simulink model "BEVplantModel"  (R2022b)
settings: Solver=daessc  StartTime=0  StopTime=50  RelTol=1e-3
PreLoadFcn:
  | % Load all parameters
  | BEVplantModelParam;
undefined symbols (not defined in the file): battery, cabin_T_init, coolant_pipe_D, coolant_valve_D_ratio_max, coolant_valve_D_ratio_min, coolant_valve_displacement, electricDrive, max_torque, vehicle, vehicleThermal
libraries: fl_lib x292, nesl_utility x67, SimscapeFluids_lib x15, ee_lib x11, sdl_lib x8, BatteryCurrentManagement x3, slpidlib x3, simulink x2, BatteryThermalManagement x1, autolibshared x1
(part 6 of 10)

== system BEVplantModel/Vehicle/Front Motor (EM1)/Inverter Power Module Thermal ==
  PM Cauer thermall : Subsystem
      settings: PortSchema="{\"entries\":[{\"content\":{\"sides\":[{\"content\":{\"connectorIds\":[\"LConn1\",\"Out1\",\"Out2\"]},\"type\":\"ConnectorPlacement.EquallySpacedRectSide\",\"uuid\":\"c466717f-a559-4c42-b6dd-2de508982627\"},{\"content\":{\"connectorIds\":[\"RConn1\",\"RConn2\"],\"side\":\"RIGHT\"},\"type\":\"ConnectorPlacement.EquallySpacedRectSide\",\"uuid\":\"5a44429a-0c01-47a4-96c4-89a03d92af2a\"},{\"content\":{\"connectorIds\":[],\"side\":\"TOP\"},\"type\":\"ConnectorPlacement.EquallySpacedRectSide\",\"uuid\":\"592797f6-2176-45a1-8a5a-ffba72eaaa30\"},{\"content\":{\"connectorIds\":[\"RConn3\"],\"side\":\"BOTTOM\"},\"type\":\"ConnectorPlacement.EquallySpacedRectSide\",\"uuid\":\"45f39216-5c54-48d4-857b-159bfbffda40\"}]},\"type\":\"ConnectorPlacement.EquallySpacedConnector\",\"uuid\":\"8211d252-7bec-4c59-be39-60a0fcf206ce\"}],\"packageUris\":[\"http://schema.mathworks.com/mf0/Connector/R2020b\"],\"version\":\"1.0\"}"
  PS Lookup Table (3D)1 : fl_lib/Physical Signals/Lookup Tables/PS Lookup Table (3D)  x1=electricDrive.loss_maps.spMat rpm  x2=electricDrive.loss_maps.tqMat N*m  x3=[25,125, 175]+273.15 K  f=electricDrive.loss_maps_inv.lossMatIgbt  interp_method=simscape.enum.interpolation.linear  extrap_method=simscape.enum.extrapolation.linear
      settings: InternalSimscapePortConfiguration="{\"Bottom\":[],\"Left\":[{\"id\":\"I1\",\"label\":\"x1\",\"type\":\"input\"},{\"id\":\"I2\",\"label\":\"x2\",\"type\":\"input\"},{\"id\":\"I3\",\"label\":\"x3\",\"type\":\"input\"}],\"Right\":[{\"id\":\"O\",\"label\":\"f\",\"type\":\"output\"}],\"Top\":[]}"
  PS Lookup Table (3D)2 : fl_lib/Physical Signals/Lookup Tables/PS Lookup Table (3D)  x1=electricDrive.loss_maps.spMat rpm  x2=electricDrive.loss_maps.tqMat N*m  x3=[25,125, 175]+273.15 K  f=electricDrive.loss_maps_inv.lossMatDiode  interp_method=simscape.enum.interpolation.linear  extrap_method=simscape.enum.extrapolation.linear
      settings: InternalSimscapePortConfiguration="{\"Bottom\":[],\"Left\":[{\"id\":\"I1\",\"label\":\"x1\",\"type\":\"input\"},{\"id\":\"I2\",\"label\":\"x2\",\"type\":\"input\"},{\"id\":\"I3\",\"label\":\"x3\",\"type\":\"input\"}],\"Right\":[{\"id\":\"O\",\"label\":\"f\",\"type\":\"output\"}],\"Top\":[]}"
  Simulink-PS Converter : nesl_utility/Simulink-PS Converter  PhysicalDomain=network_engine_domain  SubClassName=ps_input  LeftPortType=input  RightPortType=output  PseudoPeriodic=off  Frequencies=[]  NoiseDistribution=none  NoiseParameters=[]  Unit=K  AffineConversion=off  FilteringAndDerivatives=provide  SimscapeFilterOrder=1  InputFilterTimeConstant=0.001  UdotUserProvided=0
  Simulink-PS Converter1 : nesl_utility/Simulink-PS Converter  PhysicalDomain=network_engine_domain  SubClassName=ps_input  LeftPortType=input  RightPortType=output  PseudoPeriodic=off  Frequencies=[]  NoiseDistribution=none  NoiseParameters=[]  Unit=K  AffineConversion=off  FilteringAndDerivatives=provide  SimscapeFilterOrder=1  InputFilterTimeConstant=0.001  UdotUserProvided=0
  Vliq : PMIOPort  Side=Left
  Motor RPM : PMIOPort  Port=2  Side=Left
  Motor Torque : PMIOPort  Port=3  Side=Left
  H : PMIOPort  Port=4  Side=Right
  wires:
  PM Cauer thermall/1(IGBT) -> [Tigbt]
  PM Cauer thermall/2(Diode) -> [Tdiode]
  [Tdiode] -> Simulink-PS Converter1/1
  [Tigbt] -> Simulink-PS Converter/1
  connections:
  H/RConn1 -- PM Cauer thermall/LConn1
  PS Lookup Table (3D)1/RConn1 -- PM Cauer thermall/RConn2
  PS Lookup Table (3D)2/RConn1 -- PM Cauer thermall/RConn1
  Vliq/RConn1 -- PM Cauer thermall/RConn3
  Motor RPM/RConn1 -- PS Lookup Table (3D)1/LConn1 -- PS Lookup Table (3D)2/LConn1
  Motor Torque/RConn1 -- PS Lookup Table (3D)1/LConn2 -- PS Lookup Table (3D)2/LConn2
  Simulink-PS Converter1/RConn1 -- PS Lookup Table (3D)2/LConn3
  Simulink-PS Converter/RConn1 -- PS Lookup Table (3D)1/LConn3

== system BEVplantModel/Vehicle/Front Motor (EM1)/SC1 ==
  Absolute Reference (TL) : fl_lib/Thermal Liquid/Elements/Absolute Reference (TL)
  Pressure & Temperature Sensor (TL) : fl_lib/Thermal Liquid/Sensors/Pressure & Temperature Sensor (TL)
      settings: InternalSimscapePortConfiguration="{\"Bottom\":[],\"Left\":[{\"id\":\"A\",\"label\":\"A\",\"type\":\"foundation.thermal_liquid.thermal_liquid\"}],\"Right\":[{\"id\":\"B\",\"label\":\"B\",\"type\":\"foundation.thermal_liquid.thermal_liquid\"},{\"id\":\"P\",\"label\":\"P\",\"type\":\"output\"},{\"id\":\"T\",\"label\":\"T\",\"type\":\"output\"}],\"Top\":[]}"
  Volumetric Flow Rate Sensor (TL) : fl_lib/Thermal Liquid/Sensors/Volumetric Flow Rate Sensor (TL)
      settings: InternalSimscapePortConfiguration="{\"Bottom\":[],\"Left\":[{\"id\":\"A\",\"label\":\"A\",\"type\":\"foundation.thermal_liquid.thermal_liquid\"}],\"Right\":[{\"id\":\"B\",\"label\":\"B\",\"type\":\"foundation.thermal_liquid.thermal_liquid\"},{\"id\":\"V\",\"label\":\"V\",\"type\":\"output\"}],\"Top\":[]}"
  B : PMIOPort  Side=Left
  A : PMIOPort  Port=2  Side=Right
  m3/s : PMIOPort  Port=3  Side=Right
  connections:
  Pressure & Temperature Sensor (TL)/LConn1 -- Volumetric Flow Rate Sensor (TL)/RConn1 -- A/RConn1
  Volumetric Flow Rate Sensor (TL)/LConn1 -- B/RConn1
  Absolute Reference (TL)/LConn1 -- Pressure & Temperature Sensor (TL)/RConn1
  Volumetric Flow Rate Sensor (TL)/RConn2 -- m3/s/RConn1

== system BEVplantModel/Vehicle/Front Motor (EM1)/TempSens ==
  Absolute Reference (TL) : fl_lib/Thermal Liquid/Elements/Absolute Reference (TL)
  PS-Simulink Converter7 : nesl_utility/PS-Simulink Converter  PhysicalDomain=network_engine_domain  SubClassName=ps_output  LeftPortType=input  RightPortType=output  PseudoPeriodic=off  Frequencies=[]  VectorFormat=inherit  Unit=inherit  AffineConversion=off
  Pressure & Temperature Sensor (TL) : fl_lib/Thermal Liquid/Sensors/Pressure & Temperature Sensor (TL)
      settings: InternalSimscapePortConfiguration="{\"Bottom\":[],\"Left\":[{\"id\":\"A\",\"label\":\"A\",\"type\":\"foundation.thermal_liquid.thermal_liquid\"}],\"Right\":[{\"id\":\"B\",\"label\":\"B\",\"type\":\"foundation.thermal_liquid.thermal_liquid\"},{\"id\":\"P\",\"label\":\"P\",\"type\":\"output\"},{\"id\":\"T\",\"label\":\"T\",\"type\":\"output\"}],\"Top\":[]}"
  " " : PMIOPort  Side=Left
  "  " : Outport
  wires:
  PS-Simulink Converter7/1 -> "  "/1
  connections:
  Pressure & Temperature Sensor (TL)/RConn3 -- PS-Simulink Converter7/LConn1
  Absolute Reference (TL)/LConn1 -- Pressure & Temperature Sensor (TL)/RConn1
  Pressure & Temperature Sensor (TL)/LConn1 -- " "/RConn1

== system BEVplantModel/Vehicle/Front Motor (EM1)/m3//s to m//s ==
  note: Q=Av
  Coolant Area : fl_lib/Physical Signals/Sources/PS Constant  constant=4 * pi * vehicleThermal.coolant_channel_D^2 / 4 m^2
  PS Divide : fl_lib/Physical Signals/Functions/PS Divide
  PS Saturation : fl_lib/Physical Signals/Nonlinear Operators/PS Saturation  upper_limit=10 m/s  lower_limit=1e-6 m/s
  "  " : PMIOPort  Side=Left
  Vliq : PMIOPort  Port=2  Side=Right
  connections:
  PS Divide/LConn2 -- Coolant Area/RConn1
  "  "/RConn1 -- PS Divide/LConn1
  PS Divide/RConn1 -- PS Saturation/LConn1
  PS Saturation/RConn1 -- Vliq/RConn1

== system BEVplantModel/Vehicle/HVAC/Cabin ==
  Tenv : Inport
  Tsetpoint : Inport  Port=2
  acOnOff : Inport  Port=3
  HVAC Control : Subsystem
  HVAC Plant : Subsystem
  Cool : Outport
  PTC : Outport  Port=2
  wires:
  HVAC Plant/1(ptcTp) -> [Tptc]
  HVAC Control/2(PTC) -> PTC/1, HVAC Plant/3(cmdPTC)
  HVAC Control/1(cmdBlower) -> HVAC Plant/2(cmdBlower)
  HVAC Plant/2(CoolerTp) -> [TacVent]
  HVAC Plant/3(cabinTp) -> [Tcabin]
  [Tptc] -> HVAC Control/2(Tptc)
  HVAC Control/3(cmdCool) -> HVAC Plant/4(cmdCool), Cool/1
  [TacVent] -> HVAC Control/4(TacVent)
  [Tcabin] -> HVAC Control/3(Tcabin)
  Tsetpoint/1 -> HVAC Control/5(Tsetpoint)
  Tenv/1 -> HVAC Control/1(Tenv), HVAC Plant/1(EnvTp)
  acOnOff/1 -> HVAC Control/6(acOnOff)

== system BEVplantModel/Vehicle/HVAC/HVAC Demand ==
  No current : fl_lib/Physical Signals/Sources/PS Constant  constant=0 A
  PS Abs : fl_lib/Physical Signals/Nonlinear Operators/PS Abs
      settings: InternalSimscapePortConfiguration="{\"Bottom\":[],\"Left\":[{\"id\":\"I\",\"label\":\"\",\"type\":\"input\"}],\"Right\":[{\"id\":\"O\",\"label\":\"\",\"type\":\"output\"}],\"Top\":[]}"
  PS Add : fl_lib/Physical Signals/Functions/PS Add
  PS Add1 : fl_lib/Physical Signals/Functions/PS Add
  PS Divide : fl_lib/Physical Signals/Functions/PS Divide
  PS Switch : fl_lib/Physical Signals/Nonlinear Operators/PS Switch  Threshold=0.5
      settings: InternalSimscapePortConfiguration="{\"Bottom\":[],\"Left\":[{\"id\":\"I1\",\"label\":\"\",\"type\":\"input\"},{\"id\":\"I2\",\"label\":\"\",\"type\":\"input\"},{\"id\":\"I3\",\"label\":\"\",\"type\":\"input\"}],\"Right\":[{\"id\":\"O\",\"label\":\"\",\"type\":\"output\"}],\"Top\":[]}"
  Zero Divide Protection : fl_lib/Physical Signals/Sources/PS Constant  constant=1 V
  Volt : PMIOPort  Side=Left
  BatSt : PMIOPort  Port=2  Side=Left
  Cool : PMIOPort  Port=3  Side=Left
  I : PMIOPort  Port=4  Side=Right
  PTC : PMIOPort  Port=5  Side=Left
  connections:
  No current/RConn1 -- PS Switch/LConn3
  PS Add1/LConn1 -- Volt/RConn1
  PS Switch/LConn1 -- PS Divide/RConn1
  BatSt/RConn1 -- PS Switch/LConn2
  PS Switch/RConn1 -- I/RConn1
  PS Add1/RConn1 -- PS Divide/LConn2
  PS Add1/LConn2 -- Zero Divide Protection/RConn1
  PS Abs/RConn1 -- PS Add/LConn1
  Cool/RConn1 -- PS Abs/LConn1
  PTC/RConn1 -- PS Add/LConn2
  PS Add/RConn1 -- PS Divide/LConn1

== system BEVplantModel/Vehicle/HVAC/HVAC Energy ==
  I : Inport
  Batt : Inport  Port=2
  Bus Selector : BusSelector  OutputSignals=BattSensor.BatVolt
  Constant : Constant  Value=3600
  Divide : Product  Inputs=*/
  Integrator : Integrator
  Product : Product
  E : Outport
  wires:
  I/1 -> Product/1
  Divide/1 -> E/1
  Batt/1 -> Bus Selector/1
  Constant/1 -> Divide/2
  Integrator/1 -> Divide/1
  Product/1 -> Integrator/1
  Bus Selector/1 -> Product/2  "<BatVolt>"

== system BEVplantModel/Vehicle/Heater/Heater Subsystem ==
  Batt : Inport
  ThCtrl : Inport  Port=2
  Compare To Constant : simulink/Logic and Bit Operations/Compare To Constant  relop=>  const=0  OutDataTypeStr=boolean
  Heater Demand : Subsystem
  Max Power [W] : Gain  Gain=vehicleThermal.heaterMaxPower
  Product : Product
  Simulink-PS Converter : nesl_utility/Simulink-PS Converter  PhysicalDomain=network_engine_domain  SubClassName=ps_input  LeftPortType=input  RightPortType=output  PseudoPeriodic=off  Frequencies=[]  NoiseDistribution=none  NoiseParameters=[]  Unit=W  AffineConversion=off  FilteringAndDerivatives=provide  SimscapeFilterOrder=1  InputFilterTimeConstant=0.001  UdotUserProvided=0
  Simulink-PS Converter2 : nesl_utility/Simulink-PS Converter  PhysicalDomain=network_engine_domain  SubClassName=ps_input  LeftPortType=input  RightPortType=output  PseudoPeriodic=off  Frequencies=[]  NoiseDistribution=none  NoiseParameters=[]  Unit=1  AffineConversion=off  FilteringAndDerivatives=provide  SimscapeFilterOrder=1  InputFilterTimeConstant=0.001  UdotUserProvided=0
  Transfer Fcn : TransferFcn  Denominator=[1 1]
  V : PMIOPort  Side=Left
  I : PMIOPort  Port=2  Side=Right
  output : PMIOPort  Port=3  Side=Right
  wires:
  Product/1 -> Simulink-PS Converter/1
  Transfer Fcn/1 -> Max Power [W]/1
  Max Power [W]/1 -> Product/2
  Compare To Constant/1 -> Product/1
  ThCtrl/1 -> Transfer Fcn/1
  Batt/1 -> Compare To Constant/1, Simulink-PS Converter2/1
  connections:
  Simulink-PS Converter/RConn1 -- Heater Demand/LConn3 -- output/RConn1
  Heater Demand/LConn1 -- V/RConn1
  Heater Demand/LConn2 -- Simulink-PS Converter2/RConn1
  Heater Demand/RConn1 -- I/RConn1

== system BEVplantModel/Vehicle/Heater/current sensing1 ==
  Current Sensor : fl_lib/Electrical/Electrical Sensors/Current Sensor
  PS-Simulink Converter : nesl_utility/PS-Simulink Converter  PhysicalDomain=network_engine_domain  SubClassName=ps_output  LeftPortType=input  RightPortType=output  PseudoPeriodic=off  Frequencies=[]  VectorFormat=inherit  Unit=inherit  AffineConversion=off
  "  " : PMIOPort  Side=Left
  " " : PMIOPort  Port=2  Side=Right
  "   " : Outport
  wires:
  PS-Simulink Converter/1 -> "   "/1
  connections:
  PS-Simulink Converter/LConn1 -- Current Sensor/RConn1
  Current Sensor/LConn1 -- "  "/RConn1
  Current Sensor/RConn2 -- " "/RConn1

== system BEVplantModel/Vehicle/Motor Pump/Pump Demand ==
  No current : fl_lib/Physical Signals/Sources/PS Constant  constant=0 A
  PS Abs : fl_lib/Physical Signals/Nonlinear Operators/PS Abs
      settings: InternalSimscapePortConfiguration="{\"Bottom\":[],\"Left\":[{\"id\":\"I\",\"label\":\"\",\"type\":\"input\"}],\"Right\":[{\"id\":\"O\",\"label\":\"\",\"type\":\"output\"}],\"Top\":[]}"
  PS Divide : fl_lib/Physical Signals/Functions/PS Divide
  PS Product : fl_lib/Physical Signals/Functions/PS Product
  PS Switch : fl_lib/Physical Signals/Nonlinear Operators/PS Switch  Threshold=0.5
      settings: InternalSimscapePortConfiguration="{\"Bottom\":[],\"Left\":[{\"id\":\"I1\",\"label\":\"\",\"type\":\"input\"},{\"id\":\"I2\",\"label\":\"\",\"type\":\"input\"},{\"id\":\"I3\",\"label\":\"\",\"type\":\"input\"}],\"Right\":[{\"id\":\"O\",\"label\":\"\",\"type\":\"output\"}],\"Top\":[]}"
  PS Switch1 : fl_lib/Physical Signals/Nonlinear Operators/PS Switch  Threshold=0.5
      settings: InternalSimscapePortConfiguration="{\"Bottom\":[],\"Left\":[{\"id\":\"I1\",\"label\":\"\",\"type\":\"input\"},{\"id\":\"I2\",\"label\":\"\",\"type\":\"input\"},{\"id\":\"I3\",\"label\":\"\",\"type\":\"input\"}],\"Right\":[{\"id\":\"O\",\"label\":\"\",\"type\":\"output\"}],\"Top\":[]}"
  Zero Divide Protection : fl_lib/Physical Signals/Sources/PS Constant  constant=1 V
  BatSt : PMIOPort  Side=Left
  Volt : PMIOPort  Port=2  Side=Left
  Q : PMIOPort  Port=3  Side=Left
  P : PMIOPort  Port=4  Side=Left
  I : PMIOPort  Port=5  Side=Right
  connections:
  No current/RConn1 -- PS Switch/LConn3
  PS Switch1/LConn1 -- Volt/RConn1
  PS Switch/LConn1 -- PS Divide/RConn1
  BatSt/RConn1 -- PS Switch1/LConn2 -- PS Switch/LConn2
  PS Switch/RConn1 -- I/RConn1
  PS Divide/LConn1 -- PS Product/RConn1
  PS Abs/RConn1 -- PS Product/LConn2
  Q/RConn1 -- PS Product/LConn1
  P/RConn1 -- PS Abs/LConn1
  PS Switch1/RConn1 -- PS Divide/LConn2
  Zero Divide Protection/RConn1 -- PS Switch1/LConn3

== system BEVplantModel/Vehicle/Motor Pump/current sensing1 ==
  Current Sensor : fl_lib/Electrical/Electrical Sensors/Current Sensor
  PS-Simulink Converter : nesl_utility/PS-Simulink Converter  PhysicalDomain=network_engine_domain  SubClassName=ps_output  LeftPortType=input  RightPortType=output  PseudoPeriodic=off  Frequencies=[]  VectorFormat=inherit  Unit=inherit  AffineConversion=off
  "  " : PMIOPort  Side=Left
  " " : PMIOPort  Port=2  Side=Right
  "   " : Outport
  wires:
  PS-Simulink Converter/1 -> "   "/1
  connections:
  PS-Simulink Converter/LConn1 -- Current Sensor/RConn1
  Current Sensor/LConn1 -- "  "/RConn1
  Current Sensor/RConn2 -- " "/RConn1

== system BEVplantModel/Vehicle/Parallel-Serial Mode Valve/Battery Coolant Tank Heat Transfer ==
  Tenv : Inport
  Convective Heat Transfer : fl_lib/Thermal/Thermal Elements/Convective Heat Transfer  thermal_type=foundation.enum.constant_variable.constant  area=3 * vehicleThermal.coolant_tank_area m^2  heat_tr_coeff=20 W/(m^2 * K)  min_heat_tr_coeff=1e-3 W/(K*m^2)  T_specify=off  T_priority=None  T=0 K  T_nominal_specify=off  T_nominal_unit=K  T_nominal_value=1  Q_specify=off  Q_priority=None  Q=0 W  Q_nominal_specify=off  Q_nominal_unit=W  Q_nominal_value=1
  Convective Heat Transfer1 : fl_lib/Thermal/Thermal Elements/Convective Heat Transfer  thermal_type=foundation.enum.constant_variable.constant  area=3 * vehicleThermal.coolant_tank_area m^2  heat_tr_coeff=20 W/(m^2 * K)  min_heat_tr_coeff=1e-3 W/(K*m^2)  T_specify=off  T_priority=None  T=0 K  T_nominal_specify=off  T_nominal_unit=K  T_nominal_value=1  Q_specify=off  Q_priority=None  Q=0 W  Q_nominal_specify=off  Q_nominal_unit=W  Q_nominal_value=1
  Environment Temperature : fl_lib/Thermal/Thermal Sources/Controlled Temperature Source
  Simulink-PS Converter : nesl_utility/Simulink-PS Converter  PhysicalDomain=network_engine_domain  SubClassName=ps_input  LeftPortType=input  RightPortType=output  PseudoPeriodic=off  Frequencies=[]  NoiseDistribution=none  NoiseParameters=[]  Unit=K  AffineConversion=on  FilteringAndDerivatives=provide  SimscapeFilterOrder=1  InputFilterTimeConstant=0.001  UdotUserProvided=0
  Thermal Reference : fl_lib/Thermal/Thermal Elements/Thermal Reference
  A : PMIOPort  Side=Left
  B : PMIOPort  Port=2  Side=Left
  wires:
  Tenv/1 -> Simulink-PS Converter/1
  connections:
  Convective Heat Transfer/RConn1 -- Convective Heat Transfer1/RConn1 -- Environment Temperature/LConn1
  Thermal Reference/LConn1 -- Environment Temperature/RConn2
  Simulink-PS Converter/RConn1 -- Environment Temperature/RConn1
  B/RConn1 -- Convective Heat Transfer1/LConn1
  Convective Heat Transfer/LConn1 -- A/RConn1

== system BEVplantModel/Vehicle/Parallel-Serial Mode Valve/Motor Coolant Tank Heat Transfer ==
  Tenv : Inport
  Convective Heat Transfer : fl_lib/Thermal/Thermal Elements/Convective Heat Transfer  thermal_type=foundation.enum.constant_variable.constant  area=3 * vehicleThermal.coolant_tank_area m^2  heat_tr_coeff=20 W/(m^2 * K)  min_heat_tr_coeff=1e-3 W/(K*m^2)  T_specify=off  T_priority=None  T=0 K  T_nominal_specify=off  T_nominal_unit=K  T_nominal_value=1  Q_specify=off  Q_priority=None  Q=0 W  Q_nominal_specify=off  Q_nominal_unit=W  Q_nominal_value=1
  Convective Heat Transfer1 : fl_lib/Thermal/Thermal Elements/Convective Heat Transfer  thermal_type=foundation.enum.constant_variable.constant  area=3 * vehicleThermal.coolant_tank_area m^2  heat_tr_coeff=20 W/(m^2 * K)  min_heat_tr_coeff=1e-3 W/(K*m^2)  T_specify=off  T_priority=None  T=0 K  T_nominal_specify=off  T_nominal_unit=K  T_nominal_value=1  Q_specify=off  Q_priority=None  Q=0 W  Q_nominal_specify=off  Q_nominal_unit=W  Q_nominal_value=1
  Environment Temperature : fl_lib/Thermal/Thermal Sources/Controlled Temperature Source
  Simulink-PS Converter : nesl_utility/Simulink-PS Converter  PhysicalDomain=network_engine_domain  SubClassName=ps_input  LeftPortType=input  RightPortType=output  PseudoPeriodic=off  Frequencies=[]  NoiseDistribution=none  NoiseParameters=[]  Unit=K  AffineConversion=on  FilteringAndDerivatives=provide  SimscapeFilterOrder=1  InputFilterTimeConstant=0.001  UdotUserProvided=0
  Thermal Reference : fl_lib/Thermal/Thermal Elements/Thermal Reference
  A : PMIOPort  Side=Right
  B : PMIOPort  Port=2  Side=Right
  wires:
  Tenv/1 -> Simulink-PS Converter/1
  connections:
  Simulink-PS Converter/RConn1 -- Environment Temperature/RConn1
  Thermal Reference/LConn1 -- Environment Temperature/RConn2
  Convective Heat Transfer/RConn1 -- Environment Temperature/LConn1 -- Convective Heat Transfer1/RConn1
  B/RConn1 -- Convective Heat Transfer1/LConn1
  A/RConn1 -- Convective Heat Transfer/LConn1

== system BEVplantModel/Vehicle/Parallel-Serial Mode Valve/Valve Control ==
  Ctrl : Inport
  Bias : Bias  Bias=-1  SaturateOnIntegerOverflow=off
  Gain : Gain  Gain=2
  Max Valve Displacement [m] : Gain  Gain=vehicleThermal.coolant_valve_displacement
  Simulink-PS Converter : nesl_utility/Simulink-PS Converter  PhysicalDomain=network_engine_domain  SubClassName=ps_input  LeftPortType=input  RightPortType=output  PseudoPeriodic=off  Frequencies=[]  NoiseDistribution=none  NoiseParameters=[]  Unit=m  AffineConversion=off  FilteringAndDerivatives=provide  SimscapeFilterOrder=1  InputFilterTimeConstant=0.001  UdotUserProvided=0
  Transfer Fcn : TransferFcn  Denominator=[1 1]
  disp : PMIOPort  Side=Right
  wires:
  Bias/1 -> Max Valve Displacement [m]/1
  Gain/1 -> Bias/1
  Transfer Fcn/1 -> Gain/1
  Max Valve Displacement [m]/1 -> Simulink-PS Converter/1
  Ctrl/1 -> Transfer Fcn/1
  connections:
  Simulink-PS Converter/RConn1 -- disp/RConn1

== system BEVplantModel/Vehicle/Radiator/Fan_Control ==
  VehSpd : Inport
  FanCtrl : Inport  Port=2
  Air Speed Table [m/s] : Lookup_n-D  BreakpointsForDimension1=[0 40 90 110 150 180 198]  BreakpointsForDimension2=[0 14.4]  IndexSearchMethod=Linear search  BeginIndexSearchUsingPreviousIndexResult=on  Table=[0 0.8 2.2 2.7 3.6 4.1 4.6; 1.5 2.3 3.2 3.5 4.3 4.8 5.1]'  InternalRulePriority=Speed  RndMeth=Simplest
      settings: InputPortMap=u0,u1
  Fan Area [m^2] : Gain  Gain=vehicleThermal.fan_area
  Max Fan : Gain  Gain=14.4
  Simulink-PS Converter4 : nesl_utility/Simulink-PS Converter  PhysicalDomain=network_engine_domain  SubClassName=ps_input  LeftPortType=input  RightPortType=output  PseudoPeriodic=off  Frequencies=[]  NoiseDistribution=none  NoiseParameters=[]  Unit=m^3/s  AffineConversion=off  FilteringAndDerivatives=provide  SimscapeFilterOrder=1  InputFilterTimeConstant=0.001  UdotUserProvided=0
  Transfer Fcn : TransferFcn  Denominator=[5 1]
  disp : PMIOPort  Side=Right
  wires:
  Fan Area [m^2]/1 -> Simulink-PS Converter4/1
  VehSpd/1 -> Air Speed Table [m/s]/1
  FanCtrl/1 -> Max Fan/1
  Air Speed Table [m/s]/1 -> Transfer Fcn/1
  Transfer Fcn/1 -> Fan Area [m^2]/1
  Max Fan/1 -> Air Speed Table [m/s]/2
  connections:
  disp/RConn1 -- Simulink-PS Converter4/RConn1

== system BEVplantModel/Vehicle/Radiator/Subsystem ==
  s : Inport
  Bus Selector : BusSelector  OutputSignals=Env,VehSpd,cmdFan
  Bus Selector1 : BusSelector  OutputSignals=Tenv,Penv,RHenv,CO2env
  T : Outport
  p : Outport  Port=2
  RH : Outport  Port=3
  CO2 : Outport  Port=4
  VehSpd : Outport  Port=5
  cmdFan : Outport  Port=6
  wires:
  Bus Selector1/3 -> RH/1  "<RHenv>"
  Bus Selector/3 -> cmdFan/1  "<cmdFan>"
  Bus Selector/1 -> Bus Selector1/1  "<Env>"
  Bus Selector1/2 -> p/1  "<Penv>"
  s/1 -> Bus Selector/1
  Bus Selector1/1 -> T/1  "<Tenv>"
  Bus Selector/2 -> VehSpd/1  "<VehSpd>"
  Bus Selector1/4 -> CO2/1  "<CO2env>"

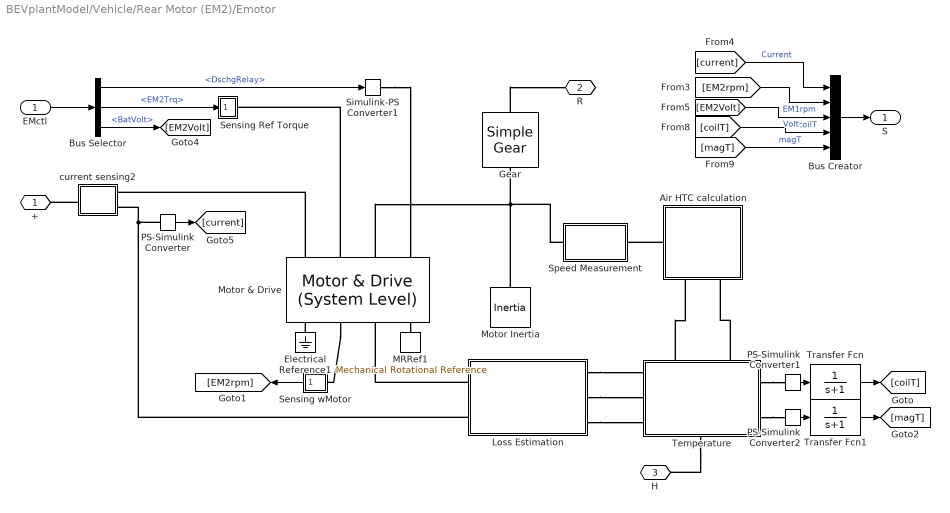
== system BEVplantModel/Vehicle/Rear Motor (EM2)/Emotor ==
  EMctl : Inport
  Air HTC calculation : Subsystem
      settings: PortSchema="{\"entries\":[{\"content\":{\"sides\":[{\"content\":{\"connectorIds\":[\"LConn1\"]},\"type\":\"ConnectorPlacement.EquallySpacedRectSide\",\"uuid\":\"c3fc49c2-0151-484f-b0d8-f4e4a060bcaf\"},{\"content\":{\"connectorIds\":[],\"side\":\"RIGHT\"},\"type\":\"ConnectorPlacement.EquallySpacedRectSide\",\"uuid\":\"c73251fe-fcad-4c5f-9d27-fb7ac98c9b31\"},{\"content\":{\"connectorIds\":[],\"side\":\"TOP\"},\"type\":\"ConnectorPlacement.EquallySpacedRectSide\",\"uuid\":\"06ea8515-c1b4-4445-9ea2-9a6fe3b8d822\"},{\"content\":{\"connectorIds\":[\"RConn1\",\"RConn2\"],\"side\":\"BOTTOM\"},\"type\":\"ConnectorPlacement.EquallySpacedRectSide\",\"uuid\":\"0d77474d-64a7-49ab-b2b5-eb3962b26dfa\"}]},\"type\":\"ConnectorPlacement.EquallySpacedConnector\",\"uuid\":\"651eda7a-2416-4496-9b8b-1b2d725cf6dd\"}],\"packageUris\":[\"http://schema.mathworks.com/mf0/Connector/R2020b\"],\"version\":\"1.0\"}"
  Bus Creator : BusCreator  Inputs=5
  Bus Selector : BusSelector  OutputSignals=DschgRelay,EM2Trq,BattSensor.BatVolt
  Electrical Reference1 : fl_lib/Electrical/Electrical Elements/Electrical Reference
  Gear : sdl_lib/Gears/Simple Gear  ratio=0.3  rotation_direction=sdl.enum.shaftOutputDirection.same  friction_model=sdl.enum.gear_efficiencies_load.off  T_noload=0.1 N*m  T_nom=5 N*m  efficiency_nom=0.8  efficiency=0.8  temperature_TLU=[280, 300, 320] K  load_TLU=[1, 5, 10] N*m  efficiency_TLU=[.95, .9, .85]  efficiency_TLU2=[.85, .8, .75; .95, .9, .85; .85, .8, .7]  w_thr=0.01 rad/s  pwr_thr=0.001 W  backlash_model=sdl.enum.backlashModel.Off  backlash_distance=1e-3 mm  x0=0 mm  r_base=0.1 m  hardstop_model=simscape.enum.hardstop.smooth  transition=1e-4 mm  backlash_stiffness=1e7 N/m  backlash_damping=1e6 N*s/m  e=0  v_tol=0.001 m/s  mu_visc=[0, 0] N*m*s/rad  enable_faults=simscape.enum.onoff.off  efficiency_fault=0.05  external_fault=simscape.enum.onoff.off  temporal_fault=simscape.enum.onoff.off  fault_time=5 s  fault_angles=pi / 12 rad  report_fault=simscape.enum.assert.action.none  thermal_mass=50 J/K  temperature_specify=off  temperature_priority=High  temperature=300 K  temperature_nominal_specify=off  temperature_nominal_unit=K  temperature_nominal_value=1  x_backlash_specify=off  x_backlash_priority=None  x_backlash=0 mm  x_backlash_nominal_specify=off  x_backlash_nominal_unit=mm  x_backlash_nominal_value=1  f_hardstop_specify=off  f_hardstop_priority=None  f_hardstop=0 N  f_hardstop_nominal_specify=off  f_hardstop_nominal_unit=N  f_hardstop_nominal_value=1  v_backlash_specify=off  v_backlash_priority=None  v_backlash=0 m/s  v_backlash_nominal_specify=off  v_backlash_nominal_unit=m/s  v_backlash_nominal_value=1
  Loss Estimation : Subsystem
  MRRef1 : fl_lib/Mechanical/Rotational Elements/Mechanical Rotational Reference
  Motor & Drive : ee_lib/Electromechanical/Motor & Drive (System Level)  torque_speed_param=2  overtorque_param=ee.enum.electromech.overtorque.no  T_t=[max_torque max_torque max_torque 0] N*m  T_t_intermittent=[.36, .32, .28, 0] N*m  T_t_2D=[.09, .09, .09; .08, .08, .08; .07, .07, .07; 0, 0, 0] N*m  T_t_intermittent_2D=[.36, .36, .36; .32, .32, .32; .28, .28, .28; 0, 0, 0] N*m  w_t=[ 0 3.75e+3 7.5e+3 8e+3 ] rpm  vdc_t=[6, 12, 24] V  torque_max=electricDrive.max_torque N*m  power_max=electricDrive.max_power W  torque_max_intermittent=0.4 N*m  power_max_intermittent=120 W  time_overtorque=30 s  time_recover=60 s  Tc=electricDrive.Tctc s  losses_param=2  eff=96  w_eff=1500 rpm  T_eff=50 N*m  Piron=200 W  Pbase=0 W  w_eff_vec=electricDrive.loss_maps.spMat rpm  T_eff_vec=electricDrive.loss_maps.tqMat N*m  v_eff_vec=[100, 250, 400] V  losses_mat=electricDrive.loss_maps.lossMat W  efficiency_mat=[95 95 95 95; 95 95 95 95; 95 95 95 95; 95 95 95 95; 95 95 95 95]  losses_mat_3D=ones(5, 4, 3) W  efficiency_mat_3D=95 * ones(5, 4, 3)  Res=0 Ohm  enable_fault=simscape.enum.onoff.on  fault_condition=1  fault_threshold=0.5  J=0 kg*m^2  lam=1e-5 N*m/(rad/s)  speed0=0 rpm  faulted_specify=off  faulted_priority=None  faulted=0  faulted_nominal_specify=off  faulted_nominal_unit=1  faulted_nominal_value=1  torqueLimitContinuous_specify=off  torqueLimitContinuous_priority=None  torqueLimitContinuous=0 N*m  torqueLimitContinuous_nominal_specify=off  torqueLimitContinuous_nominal_unit=N*m  torqueLimitContinuous_nominal_value=1  alpha=0.00393 1/K  Tmeas=30 degC  Tmeas2=31 degC  losses_mat_T2=electricDrive.loss_maps.lossMat W  efficiency_mat_T2=[95 95 95 95; 95 95 95 95; 95 95 95 95; 95 95 95 95; 95 95 95 95]  losses_mat_3D_T2=ones(5, 4, 3) W  efficiency_mat_3D_T2=95 * ones(5, 4, 3)  thermal_mass=15000 J/K  initial_temperature=vehicleThermal.coolant_T_init K
      settings: InternalSimscapePortConfiguration="{\"Bottom\":[],\"Left\":[{\"id\":\"Vp\",\"label\":\"+\",\"type\":\"foundation.electrical.electrical\"},{\"id\":\"Tr\",\"label\":\"Tr\",\"type\":\"input\"},{\"id\":\"R\",\"label\":\"R\",\"type\":\"foundation.mechanical.rotational.rotational\"},{\"id\":\"F\",\"label\":\"F\",\"type\":\"input\"}],\"Right\":[{\"id\":\"Vm\",\"label\":\"-\",\"type\":\"foundation.electrical.electrical\"},{\"id\":\"Omega\",\"label\":\"w\",\"type\":\"output\"},{\"id\":\"H\",\"label\":\"H\",\"type\":\"foundation.thermal.thermal\"},{\"id\":\"C\",\"label\":\"C\",\"type\":\"foundation.mechanical.rotational.rotational\"}],\"Top\":[]}"
  Motor Inertia : fl_lib/Mechanical/Rotational Elements/Inertia  inertia=0.02 kg*m^2  num_ports=foundation.enum.numPorts2.one  w_specify=on  w_priority=High  w=0 rpm  w_nominal_specify=off  w_nominal_unit=rad/s  w_nominal_value=1  t_specify=off  t_priority=High  t=0 N*m  t_nominal_specify=off  t_nominal_unit=N*m  t_nominal_value=1
  PS-Simulink Converter : nesl_utility/PS-Simulink Converter  PhysicalDomain=network_engine_domain  SubClassName=ps_output  LeftPortType=input  RightPortType=output  PseudoPeriodic=off  Frequencies=[]  VectorFormat=inherit  Unit=inherit  AffineConversion=off
  PS-Simulink Converter1 : nesl_utility/PS-Simulink Converter  PhysicalDomain=network_engine_domain  SubClassName=ps_output  LeftPortType=input  RightPortType=output  PseudoPeriodic=off  Frequencies=[]  VectorFormat=inherit  Unit=inherit  AffineConversion=off
  PS-Simulink Converter2 : nesl_utility/PS-Simulink Converter  PhysicalDomain=network_engine_domain  SubClassName=ps_output  LeftPortType=input  RightPortType=output  PseudoPeriodic=off  Frequencies=[]  VectorFormat=inherit  Unit=inherit  AffineConversion=off
  Sensing Ref Torque : Subsystem
  Sensing wMotor : Subsystem
      mask Display: disp('w');
  Simulink-PS Converter1 : nesl_utility/Simulink-PS Converter  PhysicalDomain=network_engine_domain  SubClassName=ps_input  LeftPortType=input  RightPortType=output  PseudoPeriodic=off  Frequencies=[]  NoiseDistribution=none  NoiseParameters=[]  Unit=1  AffineConversion=off  FilteringAndDerivatives=provide  SimscapeFilterOrder=1  InputFilterTimeConstant=0.001  UdotUserProvided=0
  Speed Measurement : Subsystem
  Temperature : Subsystem
      settings: PortSchema="{\"entries\":[{\"content\":{\"sides\":[{\"content\":{\"connectorIds\":[\"LConn1\",\"LConn2\",\"LConn3\"]},\"type\":\"ConnectorPlacement.EquallySpacedRectSide\",\"uuid\":\"fee72484-960d-4cd4-9296-e38678962aa1\"},{\"content\":{\"connectorIds\":[\"RConn1\",\"RConn2\"],\"side\":\"RIGHT\"},\"type\":\"ConnectorPlacement.EquallySpacedRectSide\",\"uuid\":\"5fc115b4-63fd-47d3-871d-1c82ac52ac43\"},{\"content\":{\"connectorIds\":[\"LConn4\",\"LConn5\"],\"side\":\"TOP\"},\"type\":\"ConnectorPlacement.EquallySpacedRectSide\",\"uuid\":\"406f719a-f995-4122-9f35-24e8332a2e84\"},{\"content\":{\"connectorIds\":[\"RConn3\"],\"side\":\"BOTTOM\"},\"type\":\"ConnectorPlacement.EquallySpacedRectSide\",\"uuid\":\"14dc85e6-8157-4b38-8651-862ce77721cd\"}]},\"type\":\"ConnectorPlacement.EquallySpacedConnector\",\"uuid\":\"1dcc2b5d-90fd-40de-873d-99118eb86bdd\"}],\"packageUris\":[\"http://schema.mathworks.com/mf0/Connector/R2020b\"],\"version\":\"1.0\"}"
  Transfer Fcn : TransferFcn  Denominator=[1 1]
  Transfer Fcn1 : TransferFcn  Denominator=[1 1]
  current sensing2 : Subsystem
  + : PMIOPort  Side=Left
  "R  " : PMIOPort  Port=2  Side=Right
  H : PMIOPort  Port=3  Side=Right
  S : Outport
  wires:
  Sensing wMotor/1(SL) -> [EM2rpm]
  [magT] -> Bus Creator/5  "magT"
  [current] -> Bus Creator/1  "Current"
  Bus Creator/1 -> S/1
  [EM2rpm] -> Bus Creator/2  "EM1rpm"
  [coilT] -> Bus Creator/4  "coilT"
  [EM2Volt] -> Bus Creator/3  "Volt"
  Bus Selector/1 -> Simulink-PS Converter1/1  "<DschgRelay>"
  Bus Selector/3 -> [EM2Volt]  "<BatVolt>"
  EMctl/1 -> Bus Selector/1
  Bus Selector/2 -> Sensing Ref Torque/1(" ")  "<EM2Trq>"
  Transfer Fcn1/1 -> [magT]
  Transfer Fcn/1 -> [coilT]
  PS-Simulink Converter1/1 -> Transfer Fcn/1
  PS-Simulink Converter2/1 -> Transfer Fcn1/1
  PS-Simulink Converter/1 -> [current]
  connections:
  Motor & Drive/RConn4 -- MRRef1/LConn1
  Motor & Drive/LConn1 -- current sensing2/RConn1
  Motor Inertia/LConn1 -- Motor & Drive/LConn3 -- Speed Measurement/LConn1 -- Gear/RConn1
  Gear/LConn1 -- "R  "/RConn1
  current sensing2/LConn1 -- +/RConn1
  Temperature/RConn3 -- H/RConn1
  Motor & Drive/LConn2 -- Sensing Ref Torque/RConn1
  Motor & Drive/RConn2 -- Sensing wMotor/LConn1
  Air HTC calculation/LConn1 -- Speed Measurement/RConn1
  Electrical Reference1/LConn1 -- Motor & Drive/RConn1
  Simulink-PS Converter1/RConn1 -- Motor & Drive/LConn4
  Loss Estimation/RConn2 -- Temperature/LConn2
  Temperature/RConn1 -- PS-Simulink Converter1/LConn1
  Temperature/RConn2 -- PS-Simulink Converter2/LConn1
  Temperature/LConn5 -- Air HTC calculation/RConn2
  Temperature/LConn4 -- Air HTC calculation/RConn1
  Loss Estimation/RConn3 -- Temperature/LConn3
  Loss Estimation/RConn1 -- Temperature/LConn1
  PS-Simulink Converter/LConn1 -- Loss Estimation/LConn2 -- current sensing2/RConn2
  Loss Estimation/LConn1 -- Motor & Drive/RConn3

== system BEVplantModel/Vehicle/Rear Motor (EM2)/Emotor Input ==
  TrqCmd : Inport
  " Batt" : Inport  Port=2
  Bus Creator : BusCreator  Inputs=3
  Bus Selector3 : BusSelector  OutputSignals=Relay.RelayDchg,BattSensor
  Constant : Constant
  Constant1 : Constant  Value=0
  Switch : Switch  Criteria=u2 > Threshold  SaturateOnIntegerOverflow=off  InputSameDT=off
  EMctl : Outport
  wires:
  TrqCmd/1 -> Bus Creator/1
  Switch/1 -> Bus Creator/2  "DschgRelay"
  Constant1/1 -> Switch/1
  Constant/1 -> Switch/3
  Bus Selector3/1 -> Switch/2  "<RelayDchg>"
  " Batt"/1 -> Bus Selector3/1
  Bus Creator/1 -> EMctl/1
  Bus Selector3/2 -> Bus Creator/3  "<BattSensor>"

== system BEVplantModel/Vehicle/Rear Motor (EM2)/Emotor Output ==
  S : Inport
  Bus Selector1 : BusSelector  OutputSignals=Current,Volt
  Constant : Constant  Value=3600
  Divide : Product  Inputs=*/
  Integrator : Integrator
  Product : Product
  EM2 : Outport
  E : Outport  Port=2
  wires:
  Divide/1 -> E/1  "EM2energy"
  Constant/1 -> Divide/2
  Integrator/1 -> Divide/1
  Product/1 -> Integrator/1
  S/1 -> EM2/1, Bus Selector1/1  "EM2sensor"
  Bus Selector1/2 -> Product/2  "<Volt>"
  Bus Selector1/1 -> Product/1  "<Current>"

== system BEVplantModel/Vehicle/Rear Motor (EM2)/Inverter Power Module Thermal ==
  PM Cauer thermall : Subsystem
      settings: PortSchema="{\"entries\":[{\"content\":{\"sides\":[{\"content\":{\"connectorIds\":[\"LConn1\",\"Out1\",\"Out2\"]},\"type\":\"ConnectorPlacement.EquallySpacedRectSide\",\"uuid\":\"c466717f-a559-4c42-b6dd-2de508982627\"},{\"content\":{\"connectorIds\":[\"RConn1\",\"RConn2\"],\"side\":\"RIGHT\"},\"type\":\"ConnectorPlacement.EquallySpacedRectSide\",\"uuid\":\"5a44429a-0c01-47a4-96c4-89a03d92af2a\"},{\"content\":{\"connectorIds\":[],\"side\":\"TOP\"},\"type\":\"ConnectorPlacement.EquallySpacedRectSide\",\"uuid\":\"592797f6-2176-45a1-8a5a-ffba72eaaa30\"},{\"content\":{\"connectorIds\":[\"RConn3\"],\"side\":\"BOTTOM\"},\"type\":\"ConnectorPlacement.EquallySpacedRectSide\",\"uuid\":\"45f39216-5c54-48d4-857b-159bfbffda40\"}]},\"type\":\"ConnectorPlacement.EquallySpacedConnector\",\"uuid\":\"8211d252-7bec-4c59-be39-60a0fcf206ce\"}],\"packageUris\":[\"http://schema.mathworks.com/mf0/Connector/R2020b\"],\"version\":\"1.0\"}"
  PS Lookup Table (3D)1 : fl_lib/Physical Signals/Lookup Tables/PS Lookup Table (3D)  x1=electricDrive.loss_maps.spMat rpm  x2=electricDrive.loss_maps.tqMat N*m  x3=[25,125, 175]  f=electricDrive.loss_maps_inv.lossMatIgbt  interp_method=simscape.enum.interpolation.linear  extrap_method=simscape.enum.extrapolation.linear
      settings: InternalSimscapePortConfiguration="{\"Bottom\":[],\"Left\":[{\"id\":\"I1\",\"label\":\"x1\",\"type\":\"input\"},{\"id\":\"I2\",\"label\":\"x2\",\"type\":\"input\"},{\"id\":\"I3\",\"label\":\"x3\",\"type\":\"input\"}],\"Right\":[{\"id\":\"O\",\"label\":\"f\",\"type\":\"output\"}],\"Top\":[]}"
  PS Lookup Table (3D)2 : fl_lib/Physical Signals/Lookup Tables/PS Lookup Table (3D)  x1=electricDrive.loss_maps.spMat rpm  x2=electricDrive.loss_maps.tqMat N*m  x3=[25,125, 175]  f=electricDrive.loss_maps_inv.lossMatDiode  interp_method=simscape.enum.interpolation.linear  extrap_method=simscape.enum.extrapolation.linear
      settings: InternalSimscapePortConfiguration="{\"Bottom\":[],\"Left\":[{\"id\":\"I1\",\"label\":\"x1\",\"type\":\"input\"},{\"id\":\"I2\",\"label\":\"x2\",\"type\":\"input\"},{\"id\":\"I3\",\"label\":\"x3\",\"type\":\"input\"}],\"Right\":[{\"id\":\"O\",\"label\":\"f\",\"type\":\"output\"}],\"Top\":[]}"
  Simulink-PS Converter : nesl_utility/Simulink-PS Converter  PhysicalDomain=network_engine_domain  SubClassName=ps_input  LeftPortType=input  RightPortType=output  PseudoPeriodic=off  Frequencies=[]  NoiseDistribution=none  NoiseParameters=[]  Unit=1  AffineConversion=off  FilteringAndDerivatives=provide  SimscapeFilterOrder=1  InputFilterTimeConstant=0.001  UdotUserProvided=0
  Simulink-PS Converter1 : nesl_utility/Simulink-PS Converter  PhysicalDomain=network_engine_domain  SubClassName=ps_input  LeftPortType=input  RightPortType=output  PseudoPeriodic=off  Frequencies=[]  NoiseDistribution=none  NoiseParameters=[]  Unit=1  AffineConversion=off  FilteringAndDerivatives=provide  SimscapeFilterOrder=1  InputFilterTimeConstant=0.001  UdotUserProvided=0
  Vliq : PMIOPort  Side=Left
  Motor RPM : PMIOPort  Port=2  Side=Left
  Motor Torque : PMIOPort  Port=3  Side=Left
  H : PMIOPort  Port=4  Side=Right
  wires:
  PM Cauer thermall/1(IGBT) -> [Tigbt]
  PM Cauer thermall/2(Diode) -> [Tdiode]
  [Tdiode] -> Simulink-PS Converter1/1
  [Tigbt] -> Simulink-PS Converter/1
  connections:
  H/RConn1 -- PM Cauer thermall/LConn1
  PS Lookup Table (3D)1/RConn1 -- PM Cauer thermall/RConn2
  PS Lookup Table (3D)2/RConn1 -- PM Cauer thermall/RConn1
  Vliq/RConn1 -- PM Cauer thermall/RConn3
  PS Lookup Table (3D)2/LConn1 -- Motor RPM/RConn1 -- PS Lookup Table (3D)1/LConn1
  PS Lookup Table (3D)2/LConn2 -- Motor Torque/RConn1 -- PS Lookup Table (3D)1/LConn2
  Simulink-PS Converter1/RConn1 -- PS Lookup Table (3D)2/LConn3
  Simulink-PS Converter/RConn1 -- PS Lookup Table (3D)1/LConn3

== system BEVplantModel/Vehicle/Rear Motor (EM2)/SC1 ==
  Absolute Reference (TL) : fl_lib/Thermal Liquid/Elements/Absolute Reference (TL)
  Pressure & Temperature Sensor (TL) : fl_lib/Thermal Liquid/Sensors/Pressure & Temperature Sensor (TL)
      settings: InternalSimscapePortConfiguration="{\"Bottom\":[],\"Left\":[{\"id\":\"A\",\"label\":\"A\",\"type\":\"foundation.thermal_liquid.thermal_liquid\"}],\"Right\":[{\"id\":\"B\",\"label\":\"B\",\"type\":\"foundation.thermal_liquid.thermal_liquid\"},{\"id\":\"P\",\"label\":\"P\",\"type\":\"output\"},{\"id\":\"T\",\"label\":\"T\",\"type\":\"output\"}],\"Top\":[]}"
  Volumetric Flow Rate Sensor (TL) : fl_lib/Thermal Liquid/Sensors/Volumetric Flow Rate Sensor (TL)
      settings: InternalSimscapePortConfiguration="{\"Bottom\":[],\"Left\":[{\"id\":\"A\",\"label\":\"A\",\"type\":\"foundation.thermal_liquid.thermal_liquid\"}],\"Right\":[{\"id\":\"B\",\"label\":\"B\",\"type\":\"foundation.thermal_liquid.thermal_liquid\"},{\"id\":\"V\",\"label\":\"V\",\"type\":\"output\"}],\"Top\":[]}"
  B : PMIOPort  Side=Left
  A : PMIOPort  Port=2  Side=Right
  m3/s : PMIOPort  Port=3  Side=Right
  connections:
  Pressure & Temperature Sensor (TL)/LConn1 -- A/RConn1 -- Volumetric Flow Rate Sensor (TL)/RConn1
  Volumetric Flow Rate Sensor (TL)/LConn1 -- B/RConn1
  Absolute Reference (TL)/LConn1 -- Pressure & Temperature Sensor (TL)/RConn1
  Volumetric Flow Rate Sensor (TL)/RConn2 -- m3/s/RConn1

== system BEVplantModel/Vehicle/Rear Motor (EM2)/m3//s to m//s ==
  note: Q=Av
  Coolant Area : fl_lib/Physical Signals/Sources/PS Constant  constant=4 * pi * vehicleThermal.coolant_channel_D^2 / 4 m^2
  PS Divide : fl_lib/Physical Signals/Functions/PS Divide
  PS Saturation : fl_lib/Physical Signals/Nonlinear Operators/PS Saturation  upper_limit=10 m/s  lower_limit=1e-6 m/s
  "  " : PMIOPort  Side=Left
  Vliq : PMIOPort  Port=2  Side=Right
  connections:
  PS Divide/LConn2 -- Coolant Area/RConn1
  "  "/RConn1 -- PS Divide/LConn1
  PS Saturation/RConn1 -- Vliq/RConn1
  PS Divide/RConn1 -- PS Saturation/LConn1

== system BEVplantModel/Controller/BMS/Battery Protection Logic/State Flow ==
  Bus Element In11 : Inport  PortName=StateInput  Element=Current
  Bus Element In1 : Inport  PortName=StateInput  Element=CurLmt
  Bus Element In2 : Inport  PortName=StateInput  Element=Volt
  Bus Element In4 : Inport  PortName=StateInput  Element=Tp
  Bus Element In6 : Inport  PortName=StateInput  Element=BatSoC
  Bus Element In7 : Inport  PortName=StateInput  Element=BatCmd
  Bus Element In8 : Inport  PortName=StateInput  Element=FaultReset
  Bus Creator8 : BusCreator  Inputs=5
  Bus Creator9 : BusCreator  Inputs=4
  Fault Protection : Stateflow chart  TreatAsAtomicUnit=on
      settings: PortSchema="{\"entries\":[{\"content\":{\"sides\":[{\"content\":{\"connectorIds\":[\"In1\",\"In2\",\"In3\",\"In4\",\"In5\",\"In6\",\"In7\"]},\"type\":\"ConnectorPlacement.EquallySpacedRectSide\",\"uuid\":\"7222f55a-2aef-4ca8-adbd-e86ed030f82f\"},{\"content\":{\"connectorIds\":[\"Out5\",\"Out6\",\"Out10\",\"Out9\",\"Out4\",\"Out1\",\"Out2\",\"Out3\",\"Out7\",\"Out8\"],\"side\":\"RIGHT\"},\"type\":\"ConnectorPlacement.EquallySpacedRectSide\",\"uuid\":\"bfa2f4e3-3563-4466-8725-57bf2336ec66\"},{\"content\":{\"connectorIds\":[],\"side\":\"TOP\"},\"type\":\"ConnectorPlacement.EquallySpacedRectSide\",\"uuid\":\"7b1e9a44-7135-4c45-bb2b-0152be29b46d\"}]},\"type\":\"ConnectorPlacement.EquallySpacedConnector\",\"uuid\":\"80032a24-3823-40c6-b797-ffbc29f7d345\"}],\"packageUris\":[\"http://schema.mathworks.com/mf0/Connector/R2020b\"],\"version\":\"1.0\"}"
  Out Bus Element : Outport  PortName=StateOut  Element=RelayRq
  Out Bus Element1 : Outport  PortName=StateOut  Element=BatSt
  Out Bus Element2 : Outport  PortName=StateOut  Element=Fault
  wires:
  Fault Protection/4(BatSt) -> Out Bus Element1/1  "BatSt"
  Fault Protection/9(RelChg) -> Bus Creator9/4  "RelayChg"
  Fault Protection/10(RelDchg) -> Bus Creator9/3  "RelayDchg"
  Fault Protection/6(Rneg) -> Bus Creator9/2  "RelayNeg"
  Fault Protection/5(Rpos) -> Bus Creator9/1  "RelayPos"
  Bus Element In7/1 -> Fault Protection/6(BatCmd)
  Bus Element In8/1 -> Fault Protection/7(FaultReset)
  Bus Element In2/1 -> Fault Protection/3(Volt)
  Bus Element In1/1 -> Fault Protection/2(CurLmt)
  Bus Element In11/1 -> Fault Protection/1(I)
  Bus Element In4/1 -> Fault Protection/4(Tp)
  Bus Element In6/1 -> Fault Protection/5(BatSoC)
  Bus Creator9/1 -> Out Bus Element/1  "RelayRq"
  Bus Creator8/1 -> Out Bus Element2/1  "Fault"
  Fault Protection/2(FaultElec) -> Bus Creator8/2  "FaultElec"
  Fault Protection/3(FaultTh) -> Bus Creator8/3  "FaultTh"
  Fault Protection/7(FaultVolt) -> Bus Creator8/4  "FaultVolt"
  Fault Protection/8(FaultDisp) -> Bus Creator8/5  "FaultDisp"
  Fault Protection/1(FaultDet) -> Bus Creator8/1  "FaultDet"

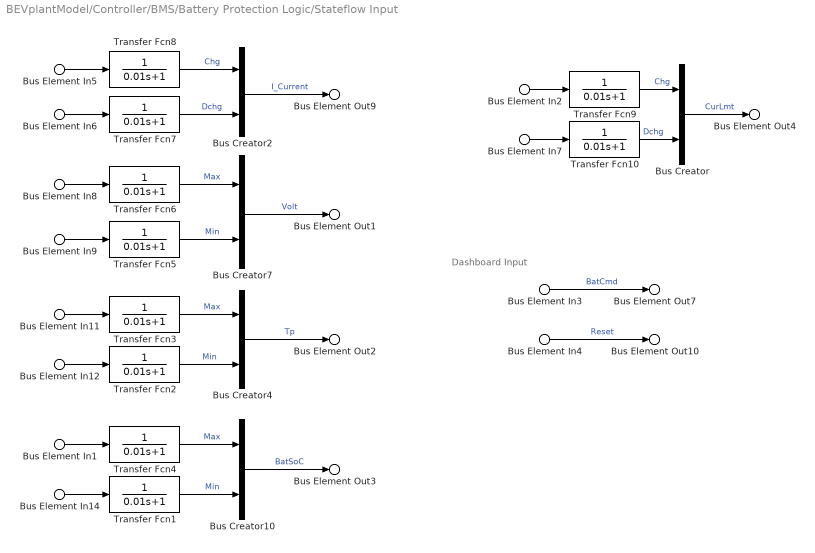
== system BEVplantModel/Controller/BMS/Battery Protection Logic/Stateflow Input ==
  note: Dashboard Input
  Bus Element In1 : Inport  PortName=SoC  Element=CellSoCmax
  Bus Element In14 : Inport  PortName=SoC  Element=CellSoCmin
  Bus Element In2 : Inport  Port=2  PortName=Current  Element=CurChgLmt
  Bus Element In7 : Inport  Port=2  PortName=Current  Element=CurDchLmt
  Bus Element In5 : Inport  Port=2  PortName=Current  Element=CurChgDchg.Chg
  Bus Element In6 : Inport  Port=2  PortName=Current  Element=CurChgDchg.Dchg
  Bus Element In8 : Inport  Port=3  PortName=Sensor  Element=CellVoltMax
  Bus Element In9 : Inport  Port=3  PortName=Sensor  Element=CellVoltMin
  Bus Element In11 : Inport  Port=3  PortName=Sensor  Element=CellTempMax
  Bus Element In12 : Inport  Port=3  PortName=Sensor  Element=CellTempMin
  Bus Element In3 : Inport  Port=3  PortName=Sensor  Element=BatCmd
  Bus Element In4 : Inport  Port=3  PortName=Sensor  Element=Reset
  Bus Creator : BusCreator  Inputs=2  OutDataTypeStr=Bus: I_Current
  Bus Creator10 : BusCreator  Inputs=2  OutDataTypeStr=Bus: MaxMinLimit
  Bus Creator2 : BusCreator  Inputs=2  OutDataTypeStr=Bus: I_Current
  Bus Creator4 : BusCreator  Inputs=2  OutDataTypeStr=Bus: MaxMinLimit
  Bus Creator7 : BusCreator  Inputs=2  OutDataTypeStr=Bus: CellVoltage  NonVirtualBus=on
  Transfer Fcn{1..10} (10 alike) : TransferFcn  Denominator=[0.01 1]
  Bus Element Out9 : Outport  PortName=StateInput  Element=Current
  Bus Element Out1 : Outport  PortName=StateInput  Element=Volt
  Bus Element Out2 : Outport  PortName=StateInput  Element=Tp
  Bus Element Out3 : Outport  PortName=StateInput  Element=BatSoC
  Bus Element Out4 : Outport  PortName=StateInput  Element=CurLmt
  Bus Element Out7 : Outport  PortName=StateInput  Element=BatCmd
  Bus Element Out10 : Outport  PortName=StateInput  Element=FaultReset
  wires:
  Transfer Fcn10/1 -> Bus Creator/2  "Dchg"
  Transfer Fcn9/1 -> Bus Creator/1  "Chg"
  Transfer Fcn7/1 -> Bus Creator2/2  "Dchg"
  Transfer Fcn8/1 -> Bus Creator2/1  "Chg"
  Transfer Fcn6/1 -> Bus Creator7/1  "Max"
  Transfer Fcn5/1 -> Bus Creator7/2  "Min"
  Transfer Fcn3/1 -> Bus Creator4/1  "Max"
  Transfer Fcn2/1 -> Bus Creator4/2  "Min"
  Transfer Fcn1/1 -> Bus Creator10/2  "Min"
  Transfer Fcn4/1 -> Bus Creator10/1  "Max"
  Bus Element In7/1 -> Transfer Fcn10/1
  Bus Element In2/1 -> Transfer Fcn9/1
  Bus Creator7/1 -> Bus Element Out1/1  "Volt"
  Bus Creator2/1 -> Bus Element Out9/1  "I_Current"
  Bus Creator4/1 -> Bus Element Out2/1  "Tp"
  Bus Element In3/1 -> Bus Element Out7/1  "BatCmd"
  Bus Element In4/1 -> Bus Element Out10/1  "Reset"
  Bus Element In14/1 -> Transfer Fcn1/1
  Bus Element In1/1 -> Transfer Fcn4/1
  Bus Element In6/1 -> Transfer Fcn7/1
  Bus Element In5/1 -> Transfer Fcn8/1
  Bus Creator10/1 -> Bus Element Out3/1  "BatSoC"
  Bus Element In11/1 -> Transfer Fcn3/1
  Bus Creator/1 -> Bus Element Out4/1  "CurLmt"
  Bus Element In9/1 -> Transfer Fcn5/1
  Bus Element In8/1 -> Transfer Fcn6/1
  Bus Element In12/1 -> Transfer Fcn2/1

== system BEVplantModel/Controller/BMS/MinMax Current Limiter/Current Directional ==
  CurDir : Inport
  Cur : Inport  Port=2
  Abs : Abs  SaturateOnIntegerOverflow=off
  Bus Creator2 : BusCreator  Inputs=2  OutDataTypeStr=Bus: I_Current
  Bus Selector : BusSelector  OutputSignals=Chg,Dsch
  Gain : Gain  Gain=-1
  Product : Product
  Product1 : Product
  I_Current : Outport
  wires:
  Gain/1 -> Product/1
  Cur/1 -> Abs/1
  Abs/1 -> Product/2, Product1/2
  CurDir/1 -> Bus Selector/1
  Bus Selector/1 -> Gain/1  "<Chg>"
  Bus Selector/2 -> Product1/1  "<Dsch>"
  Product/1 -> Bus Creator2/1  "Chg"
  Bus Creator2/1 -> I_Current/1  "I_Current"
  Product1/1 -> Bus Creator2/2  "Dchg"

== system BEVplantModel/Controller/BMS/MinMax Current Limiter/OCprotection ==
  Cur : Inport
  VoltMax : Inport  Port=2
  CellTpMax : Inport  Port=3
  CellTpMin : Inport  Port=4
  Add : Sum  Inputs=-+
  ChrgCurrLimitMaxTp : Lookup_n-D  NumberOfTableDimensions=1  BreakpointsForDimension1="single([313  318  323  328 333])"  BreakpointsForDimension3=[5, 7]  Table=single([1.0 0.8 0.5 0.3 0])  ExtrapMethod=Clip  UseLastTableValue=on  InternalRulePriority=Speed  RndMeth=Simplest
  ChrgCurrLimitMinTp : Lookup_n-D  NumberOfTableDimensions=1  BreakpointsForDimension1=single([258 263 268 273 278 283 288])  BreakpointsForDimension3=[5, 7]  Table="single([0.1 0.2  0.3 0.3 0.5 1.0 1.0])"  ExtrapMethod=Clip  UseLastTableValue=on  InternalRulePriority=Speed  RndMeth=Simplest
  ChrgCurrLimitVolt : Lookup_n-D  NumberOfTableDimensions=1  BreakpointsForDimension1=single([3.9 4.0 4.15 4.2])  BreakpointsForDimension3=[5, 7]  Table="single([1.0 0.8 0.3  0.3])"  ExtrapMethod=Clip  UseLastTableValue=on  InternalRulePriority=Speed  RndMeth=Simplest
  Constant : Constant  Value=10
  MaxChrgCurLim : Gain  Gain=-battery.MaxChrgCurLim
  Min : MinMax  Inputs=3
  Np_Module : Gain  Gain=battery.Np
  Relational Operator : RelationalOperator  Operator=<=  OutDataTypeStr=boolean  RndMeth=Simplest  InputSameDT=off
  OCWarn : Outport
  ChrgCurLim : Outport  Port=2
  wires:
  Add/1 -> Relational Operator/1
  Constant/1 -> Add/1
  VoltMax/1 -> ChrgCurrLimitVolt/1
  ChrgCurrLimitVolt/1 -> Min/1  "ChrgCurrLimVolt"
  MaxChrgCurLim/1 -> Np_Module/1
  Np_Module/1 -> ChrgCurLim/1, [ChrgCurLim]  "CurChrgLmt"
  CellTpMax/1 -> ChrgCurrLimitMaxTp/1
  CellTpMin/1 -> ChrgCurrLimitMinTp/1
  ChrgCurrLimitMaxTp/1 -> Min/2  "MaxTpChrgCurrLim"
  ChrgCurrLimitMinTp/1 -> Min/3  "MinTpChrgCurrLim"
  Min/1 -> MaxChrgCurLim/1
  Cur/1 -> Relational Operator/2
  [ChrgCurLim] -> Add/2
  Relational Operator/1 -> OCWarn/1
